simulink model "ksrbl_4k4t_hdtrig"  (Simulink 6.2)
settings: Solver=ode45  StartTime=0.0  StopTime=20000  RelTol=1e-3
libraries: xbsIndex_r3 x1214, casper_library x120, xps_library x20
(part 10 of 26)

== system ksrbl_4k4t_hdtrig/pfb_fir_real/pol1_in1_first_tap/pfb_coeff_gen ==
  din : Inport  Port=1  LatchInput=off
  sync : Inport  Port=2  LatchInput=off
  Concat : xbsIndex_r3/Concat  num_inputs=4  explicit_period=off  period=1  dbl_ovrd=off
  Counter : xbsIndex_r3/Counter  cnt_type=Free Running  n_bits=10  bin_pt=0  arith_type=Unsigned  start_count=0  cnt_to=Inf  cnt_by_val=1  operation=Up  explicit_period=on  period=1  load_pin=off  rst=on  en=off  dbl_ovrd=off  show_param=off  use_rpm=on  gen_core=off
      settings: xl_area=[0, 0, 0, 0, 0, 0, 0]
  Delay : xbsIndex_r3/Delay  latency=bram_latency+1  reg_retiming=off  explicit_period=off  period=1  en=off  accept_only_valid=off  init_zero=on  dbl_ovrd=off  show_param=off
      settings: xl_area=[0, 0, 0, 0, 0, 0, 0]
  Delay1 : xbsIndex_r3/Delay  latency=5  reg_retiming=off  explicit_period=off  period=1  en=off  accept_only_valid=off  init_zero=on  dbl_ovrd=off  show_param=off
      settings: xl_area=[0, 0, 0, 0, 0, 0, 0]
  ROM1 : xbsIndex_r3/ROM  depth=1024  initVector=[-3.1185374660155e-018 -3.90817859203733e-005 -7.82029942377348e-005 -0.000117364902610826 -0.000156568791093434 -0.000195815942087653 -0.000235107640297013 -0.000274445172679356 -0.00031382982839976 -0.000353262898783155 -0.000392745677266923 -0.000432279459353376 -0.000471865542561998 -0.000511505226381663 -0.000551199812222732 -0.000590950603368917 -0.000630758904929125 -0.000670626023789185 -0.000710553268563328 -0.00075054194954573 -0.000790593378661751 -0.000830708869419183 -0.000870889736859361 -0.00091113729750808 -0.000951452869326473 -0.00099183777166179 -0.00103229332519796 -0.00107282085190612 -0.00111342167499508 -0.00115409711886151 -0.00119484850904021 -0.00123567717215412 -0.00127658443586429 -0.00131757162881981 -0.00135864008060744 -0.00139979112170133 -0.00144102608341258 -0.0014823462978386 -0.00152375309781249 -0.00156524781685233 -0.00160683178911018 -0.00164850634932128 -0.00169027283275283 -0.00173213257515293 -0.00177408691269934 -0.00181613718194805 -0.00185828471978188 -0.00190053086335898 -0.00194287695006116 -0.00198532431744216 -0.00202787430317591 -0.00207052824500455 -0.00211328748068654 -0.00215615334794452 -0.00219912718441318 -0.00224221032758705 -0.00228540411476815 -0.00232870988301357 -0.00237212896908308 -0.00241566270938644 -0.00245931243993086 -0.00250307949626824 -0.00254696521344237 -0.00259097092593612 -0.0026350979676184 -0.00267934767169121 -0.00272372137063657 -0.00276822039616328 -0.00281284607915377 -0.00285759974961077 -0.00290248273660395 -0.00294749636821646 -0.0029926419714915 -0.00303792087237869 -0.00308333439568051 -0.00312888386499854 -0.00317457060267975 -0.00322039592976276 -0.00326636116592387 -0.00331246762942315 -0.00335871663705057 -0.00340510950407184 -0.00345164754417438 -0.00349833206941318 -0.00354516439015661 -0.00359214581503217 -0.00363927765087218 -0.00368656120265948 -0.00373399777347301 -0.00378158866443341 -0.00382933517464849 -0.00387723860115878 -0.00392530023888291 -0.003973521380563 -0.00402190331671011 -0.0040704473355494 -0.00411915472296558 -0.004168026762448 -0.00421706473503593 -0.00426626991926379 -0.00431564359110616 -0.00436518702392296 -0.00441490148840456 -0.00446478825251676 -0.00451484858144581 -0.0045650837375435 -0.00461549498027197 -0.00466608356614881 -0.00471685074869185 -0.00476779777836413 -0.00481892590251875 -0.00487023636534373 -0.0049217304078068 -0.00497340926760033 -0.005025274179086 -0.00507732637323965 -0.00512956707759609 -0.00518199751619374 -0.00523461890951954 -0.00528743247445352 -0.00534043942421364 -0.00539364096830049 -0.00544703831244197 -0.00550063265853799 -0.00555442520460526 -0.00560841714472187 -0.00566260966897206 -0.00571700396339093 -0.00577160120990909 -0.00582640258629735 -0.00588140926611151 -0.00593662241863694 -0.00599204320883343 -0.00604767279727977 -0.00610351234011856 -0.00615956298900096 -0.00621582589103136 -0.00627230218871218 -0.00632899301988868 -0.00638589951769364 -0.00644302281049225 -0.00650036402182689 -0.00655792427036195 -0.00661570466982872 -0.00667370632897022 -0.00673193035148608 -0.00679037783597755 -0.00684904987589229 -0.00690794755946946 -0.00696707196968468 -0.00702642418419498 -0.00708600527528392 -0.00714581630980666 -0.00720585834913499 -0.00726613244910261 -0.00732663965995014 -0.00738738102627043 -0.00744835758695382 -0.00750957037513333 -0.00757102041813002 -0.00763270873739842 -0.00769463634847182 -0.00775680426090774 -0.00781921347823351 -0.00788186499789164 -0.00794475981118556 -0.00800789890322511 -0.00807128325287227 -0.00813491383268693 -0.00819879160887258 -0.00826291754122212 -0.00832729258306389 -0.0083919176812074 -0.00845679377588946 -0.00852192180072018 -0.00858730268262907 -0.00865293734181122 -0.00871882669167352 -0.00878497163878088 -0.00885137308280274 -0.00891803191645931 -0.00898494902546814 -0.00905212528849068 -0.00911956157707884 -0.0091872587556217 -0.00925521768129231 -0.00932343920399441 -0.00939192416630946 -0.00946067340344352 ...(+16631 chars)]  arith_type="Signed  (2's comp)"  n_bits=8  bin_pt=7  latency=4  init_zero=on  explicit_period=off  period=1  rst=off  init_reg=0  en=off  dbl_ovrd=off  show_param=on  distributed_mem=off  use_rpm=on  gen_core=off
      settings: xl_area=[0, 0, 0, 0, 0, 0, 0]
  ROM2 : xbsIndex_r3/ROM  depth=1024  initVector=[2.10518471702391e-017 0.000528591329667851 0.00105959305888785 0.00159300724253355 0.00212883591107237 0.00266708107049428 0.00320774470224115 0.00375082876313597 0.00429633518531311 0.00484426587614807 0.00539462271818799 0.00594740756908197 0.0065026222615125 0.00706026860312642 0.00762034837646618 0.00818286333890216 0.00874781522256437 0.00931520573427505 0.009885036555481 0.0104573093421871 0.0110320257248891 0.0116091873085076 0.0121887956723214 0.0127708523699021 0.0133553589290488 0.013942316851722 0.0145317276139797 0.015123592665912 0.0157179134315774 0.0163146913089384 0.016913927669798 0.0175156238597365 0.0181197811980482 0.0187264009776786 0.0193354844651624 0.0199470329005612 0.0205610474974011 0.0211775294426126 0.0217964798964683 0.0224178999925225 0.0230417908375507 0.0236681535114895 0.0242969890673768 0.0249282985312921 0.0255620829022974 0.0261983431523784 0.0268370802263863 0.0274782950419788 0.0281219884895631 0.028768161432238 0.029416814705737 0.0300679491183708 0.0307215654509716 0.0313776644568366 0.0320362468616724 0.0326973133635389 0.033360864632795 0.0340269013120434 0.0346954240160762 0.0353664333318208 0.0360399298182863 0.0367159140065104 0.0373943863995053 0.0380753474722063 0.0387587976714189 0.0394447374157666 0.0401331670956398 0.0408240870731443 0.0415174976820505 0.0422133992277424 0.0429117919871683 0.0436126762087903 0.0443160521125352 0.0450219198897449 0.0457302797031285 0.0464411316867136 0.0471544759457977 0.0478703125569017 0.0485886415677217 0.049309462997083 0.0500327768348925 0.0507585830420937 0.0514868815506202 0.0522176722633509 0.0529509550540641 0.0536867297673939 0.0544249962187857 0.0551657541944515 0.0559090034513275 0.0566547437170307 0.0574029746898158 0.0581536960385331 0.0589069074025866 0.0596626083918926 0.0604207985868383 0.0611814775382407 0.0619446447673069 0.0627102997655937 0.0634784419949678 0.0642490708875669 0.065022185845761 0.0657977862421134 0.066575871419343 0.0673564406902867 0.0681394933378623 0.068925028615031 0.0697130457447615 0.070503543919994 0.0712965223036042 0.0720919800283679 0.072889916196927 0.0736903298817541 0.074493220125119 0.0752985859390548 0.0761064263053248 0.0769167401753897 0.0777295264703751 0.0785447840810393 0.0793625118677423 0.080182708660414 0.0810053732585234 0.0818305044310489 0.0826581009164475 0.0834881614226262 0.0843206846269117 0.0851556691760228 0.0859931136860413 0.0868330167423848 0.0876753768997786 0.088520192682229 0.0893674625829969 0.0902171850645708 0.091069358558642 0.0919239814660785 0.0927810521569007 0.093640568970256 0.0945025302143957 0.0953669341666506 0.0962337790734082 0.0971030631500895 0.0979747845811271 0.0988489415199428 0.0997255320889262 0.100604554379414 0.101486006451668 0.102369886334857 0.103256192027036 0.104144921495124 0.105036072674892 0.105929643470936 0.106825631756666 0.107724035374284 0.108624852134769 0.109528079817859 0.110433716172034 0.111341758914505 0.11225220573119 0.113165054276707 0.114080302174356 0.114997947016103 0.11591798636257 0.11684041774302 0.117765238655343 0.118692446566047 0.119622038910243 0.120554013091632 0.121488366482501 0.122425096423704 0.123364200224658 0.124305675163328 0.125249518486225 0.126195727408388 0.127144299113384 0.128095230753296 0.129048519448714 0.130004162288731 0.130962156330938 0.13192249860141 0.132885186094711 0.13385021577388 0.134817584570431 0.135787289384346 0.136759327084073 0.137733694506524 0.138710388457066 0.139689405709526 0.140670743006182 0.141654397057769 0.142640364543469 0.143628642110919 0.144619226376203 0.145612113923859 0.146607301306874 0.14760478504669 0.1486045616332 0.149606627524756 0.150610979148169 0.151617612898708 0.152626525140111 0.153637712204582 0.154651170392802 0.155666895973925 0.156684885185591 0.157705134233931 0.158727639293566 0.159752396507623 0.160779401987735 0.161808651814054 0.162840142035253 0.163873868668541 0.164909827699666 0.16594801508293 0.166988426741192 0.168031058565885 ...(+14491 chars)]  arith_type="Signed  (2's comp)"  n_bits=8  bin_pt=7  latency=4  init_zero=on  explicit_period=off  period=1  rst=off  init_reg=0  en=off  dbl_ovrd=off  show_param=on  distributed_mem=off  use_rpm=on  gen_core=off
      settings: xl_area=[0, 0, 0, 0, 0, 0, 0]
  ROM3 : xbsIndex_r3/ROM  depth=1024  initVector=[0.999999991542525 0.999997746215142 0.999991280893574 0.999980595640379 0.999965690558761 0.999946565792566 0.999923221526282 0.999895657985032 0.999863875434578 0.999827874181312 0.999787654572254 0.999743216995048 0.999694561877954 0.999641689689849 0.999584600940211 0.999523296179123 0.999457775997257 0.99938804102587 0.999314091936799 0.999235929442443 0.999153554295766 0.999066967290274 0.998976169260017 0.998881161079569 0.998781943664019 0.998678517968961 0.998570884990482 0.998459045765144 0.998343001369976 0.998222752922455 0.998098301580497 0.997969648542435 0.997836795047011 0.997699742373352 0.997558491840959 0.997413044809688 0.99726340267973 0.997109566891595 0.996951538926095 0.99678932030432 0.99662291258762 0.996452317377585 0.996277536316026 0.996098571084948 0.995915423406535 0.99572809504312 0.995536587797169 0.995340903511252 0.99514104406802 0.994937011390186 0.994728807440489 0.994516434221678 0.994299893776482 0.994079188187582 0.993854319577588 0.993625290109003 0.993392101984206 0.993154757445413 0.992913258774655 0.992667608293741 0.992417808364236 0.992163861387422 0.991905769804272 0.991643536095417 0.991377162781111 0.991106652421201 0.990832007615091 0.990553231001712 0.99027032525948 0.989983293106271 0.989692137299378 0.989396860635475 0.989097465950585 0.98879395612004 0.988486334058444 0.988174602719633 0.987858765096639 0.987538824221651 0.987214783165971 0.986886645039981 0.986554412993095 0.986218090213723 0.985877679929228 0.98553318540588 0.98518460994882 0.984831956902013 0.984475229648201 0.984114431608868 0.983749566244185 0.983380637052971 0.983007647572648 0.982630601379188 0.982249502087074 0.981864353349249 0.981475158857069 0.981081922340253 0.980684647566838 0.980283338343126 0.979877998513636 0.979468631961054 0.979055242606184 0.978637834407891 0.978216411363056 0.97779097750652 0.977361536911031 0.976928093687194 0.976490651983415 0.976049215985846 0.975603789918334 0.975154378042359 0.974700984656988 0.974243614098811 0.973782270741888 0.97331695899769 0.972847683315044 0.972374448180072 0.971897258116136 0.971416117683776 0.97093103148065 0.970442004141479 0.969949040337981 0.969452144778811 0.968951322209504 0.968446577412408 0.967937915206624 0.967425340447943 0.966908858028783 0.966388472878124 0.965864189961445 0.96533601428066 0.96480395087405 0.964268004816201 0.963728181217935 0.963184485226244 0.962636922024225 0.96208549683101 0.961530214901699 0.960971081527293 0.960408102034622 0.959841281786279 0.959270626180548 0.958696140651335 0.958117830668096 0.957535701735767 0.956949759394692 0.956360009220551 0.955766456824289 0.955169107852038 0.954567967985051 0.953963042939622 0.953354338467014 0.952741860353385 0.952125614419711 0.951505606521714 0.95088184254978 0.950254328428887 0.949623070118529 0.948988073612632 0.948349344939485 0.947706890161655 0.947060715375912 0.946410826713146 0.945757230338293 0.94509993245025 0.944438939281797 0.943774257099516 0.943105892203709 0.942433850928316 0.941758139640834 0.941078764742236 0.940395732666881 0.939709049882441 0.939018722889808 0.938324758223014 0.937627162449148 0.936925942168265 0.936221104013307 0.935512654650013 0.934800600776835 0.934084949124849 0.93336570645767 0.932642879571361 0.931916475294352 0.931186500487344 0.930452962043223 0.929715866886972 0.928975221975582 0.928231034297958 0.927483310874834 0.926732058758677 0.9259772850336 0.925218996815267 0.924457201250805 0.923691905518707 0.922923116828743 0.922150842421867 0.921375089570118 0.920595865576533 0.91981317777505 0.919027033530411 0.918237440238071 0.9174444053241 0.916647936245088 0.915848040488046 0.915044725570316 0.914237999039468 0.913427868473204 0.912614341479263 0.911797425695319 0.910977128788886 0.910153458457217 0.909326422427204 0.908496028455283 0.90766228432733 0.90682519785856 0.905984776893432 0.905141029305539 0.904293962997516 0.903443585900934 0.902589905976196 0.901732931212439 0.900872669627427 0.900009129267451 ...(+14479 chars)]  arith_type="Signed  (2's comp)"  n_bits=8  bin_pt=7  latency=4  init_zero=on  explicit_period=off  period=1  rst=off  init_reg=0  en=off  dbl_ovrd=off  show_param=off  distributed_mem=off  use_rpm=on  gen_core=off
      settings: xl_area=[0, 0, 0, 0, 0, 0, 0]
  ROM4 : xbsIndex_r3/ROM  depth=1024  initVector=[2.10449700717643e-017 -0.000526010894157433 -0.00104961590983381 -0.00157081717653369 -0.00208961684787401 -0.00260601710151125 -0.00312002013906894 -0.00363162818606433 -0.00414084349183562 -0.00464766832946811 -0.00515210499572064 -0.00565415581095117 -0.00615382311904299 -0.0066511092873299 -0.00714601670652118 -0.00763854779062697 -0.00812870497688262 -0.00861649072567327 -0.00910190752045772 -0.0095849578676928 -0.0100656442967567 -0.0105439693598725 -0.0110199356320313 -0.0114935457109151 -0.0119648022168198 -0.0124337077925771 -0.0129002651034771 -0.0133644768371902 -0.0138263457036888 -0.0142858744351686 -0.0147430657859702 -0.0151979225325 -0.0156504474731507 -0.0161006434282222 -0.016548513239842 -0.016994059771885 -0.0174372859098934 -0.0178781945609966 -0.0183167886538307 -0.0187530711384574 -0.0191870449862829 -0.0196187131899773 -0.0200480787633926 -0.0204751447414813 -0.0208999141802143 -0.0213223901564992 -0.0217425757680977 -0.0221604741335434 -0.0225760883920587 -0.0229894217034722 -0.0234004772481359 -0.0238092582268408 -0.0242157678607347 -0.0246200093912377 -0.0250219860799587 -0.0254217012086108 -0.0258191580789274 -0.0262143600125781 -0.0266073103510828 -0.0269980124557283 -0.0273864697074822 -0.0277726855069081 -0.0281566632740801 -0.0285384064484972 -0.0289179184889977 -0.0292952028736727 -0.0296702630997806 -0.0300431026836605 -0.0304137251606456 -0.0307821340849767 -0.0311483330297152 -0.0315123255866565 -0.0318741153662423 -0.0322337059974734 -0.0325911011278226 -0.0329463044231465 -0.033299319567598 -0.0336501502635381 -0.033998800231448 -0.0343452732098405 -0.0346895729551718 -0.0350317032417527 -0.0353716678616599 -0.0357094706246472 -0.0360451153580562 -0.0363786059067274 -0.0367099461329104 -0.0370391399161748 -0.0373661911533205 -0.0376911037582876 -0.038013881662067 -0.0383345288126096 -0.038653049174737 -0.0389694467300506 -0.0392837254768411 -0.0395958894299981 -0.0399059426209194 -0.0402138890974202 -0.0405197329236417 -0.0408234781799606 -0.0411251289628975 -0.0414246893850255 -0.0417221635748791 -0.0420175556768622 -0.0423108698511568 -0.042602110273631 -0.0428912811357467 -0.0431783866444683 -0.0434634310221702 -0.0437464185065442 -0.0440273533505079 -0.0443062398221116 -0.0445830822044459 -0.0448578847955492 -0.0451306519083147 -0.0454013878703979 -0.0456700970241231 -0.0459367837263909 -0.0462014523485845 -0.0464641072764771 -0.0467247529101379 -0.0469833936638393 -0.047240033965963 -0.0474946782589065 -0.0477473309989893 -0.0479979966563597 -0.0482466797149003 -0.0484933846721344 -0.0487381160391319 -0.0489808783404156 -0.0492216761138665 -0.0494605139106299 -0.0496973962950215 -0.0499323278444321 -0.0501653131492341 -0.0503963568126868 -0.0506254634508413 -0.0508526376924469 -0.0510778841788556 -0.0513012075639276 -0.0515226125139367 -0.0517421037074757 -0.0519596858353606 -0.0521753636005368 -0.0523891417179833 -0.0526010249146181 -0.052811017929203 -0.0530191255122482 -0.0532253524259179 -0.0534297034439341 -0.0536321833514821 -0.0538327969451149 -0.054031549032658 -0.0542284444331139 -0.054423487976567 -0.0546166845040876 -0.0548080388676372 -0.0549975559299724 -0.0551852405645498 -0.0553710976554303 -0.0555551320971833 -0.0557373487947917 -0.0559177526635558 -0.0560963486289979 -0.0562731416267665 -0.0564481366025409 -0.0566213385119356 -0.056792752320404 -0.0569623830031435 -0.0571302355449993 -0.0572963149403688 -0.0574606261931062 -0.0576231743164263 -0.057783964332809 -0.0579430012739038 -0.0581002901804337 -0.0582558361020998 -0.0584096440974854 -0.0585617192339605 -0.0587120665875858 -0.0588606912430172 -0.0590075982934104 -0.0591527928403246 -0.0592962799936273 -0.0594380648713987 -0.0595781525998359 -0.0597165483131572 -0.0598532571535069 -0.0599882842708593 -0.0601216348229238 -0.0602533139750483 -0.0603833269001251 -0.0605116787784943 -0.060638374797849 -0.0607634201531396 -0.0608868200464788 -0.0610085796870458 -0.0611287042909915 -0.0612471990813427 ...(+16639 chars)]  arith_type="Signed  (2's comp)"  n_bits=8  bin_pt=7  latency=4  init_zero=on  explicit_period=off  period=1  rst=off  init_reg=0  en=off  dbl_ovrd=off  show_param=off  distributed_mem=off  use_rpm=on  gen_core=off
      settings: xl_area=[0, 0, 0, 0, 0, 0, 0]
  Register : xbsIndex_r3/Register  init=0  reg_only_valid=off  explicit_period=off  period=1  rst=off  en=off  out_en=off  dbl_ovrd=off  show_param=off
      settings: xl_area=[0, 0, 0, 0, 0, 0, 0]
  Reinterpret{1..4} (4 alike) : xbsIndex_r3/Reinterpret  force_arith_type=on  arith_type=Unsigned  force_bin_pt=on  bin_pt=0  force_valid=on
  dout : Outport
  sync_out : Outport  Port=2
  coeff : Outport  Port=3
  wires:
  din/1 -> Delay1/1
  Delay1/1 -> dout/1
  sync/1 -> Counter/1, Delay/1
  Delay/1 -> sync_out/1
  Concat/1 -> Register/1
  Register/1 -> coeff/1
  Counter/1 -> ROM1/1, ROM2/1, ROM3/1, ROM4/1
  ROM1/1 -> Reinterpret1/1
  Reinterpret1/1 -> Concat/1
  ROM2/1 -> Reinterpret2/1
  Reinterpret2/1 -> Concat/2
  ROM3/1 -> Reinterpret3/1
  Reinterpret3/1 -> Concat/3
  ROM4/1 -> Reinterpret4/1
  Reinterpret4/1 -> Concat/4
